simulink model "eVTOL_PX4_2023b"  (R2024b)
settings: Solver=ode4  StartTime=0  StopTime=inf  FixedStep=0.01  RelTol=1e-3
values from neighbouring files (symbols this model uses):
  aDl =     [initdata.mat]
  aDr =     [initdata.mat]
  aDyn =     [initdata.mat]
  Airport = init_airport('PHNL')    [initdata_HIL_eVTOL.m]
  aLat =     [initdata.mat]
  aLon =     [initdata.mat]
  D = Prop.D    [EOM_dt_MC.m]    (also in EOM_get_alf_dt_de_prop_evtol.m = CD * QS)
  dt0 = X(2)    [EOM_get_alf_dt_de_prop_evtol.m]    (also in initdata.mat = 0.258252593971; initdata_HIL_eVTOL.m = EOM_dt_MC)
  EAS0 = TAS0 / EAS2TAS    [initdata_HIL_eVTOL.m]
  FCS = init_FCS    [initdata_HIL_eVTOL.m]
  General = init_layoutdata    [EOM_dt_MC.m]    (also in build_optimized_CA.m; initdata.mat = ; initdata_HIL_eVTOL.m)
  h0 = Con(1)    [EOM_get_alf_dt_de_prop_evtol.m]    (also in initdata.mat = 450; initdata_HIL_eVTOL.m = 50)
  mass = Con(3)    [EOM_get_alf_dt_de_prop_evtol.m]    (also in initdata.mat = 2255.54; initdata_HIL_eVTOL.m = 7)
  Motor = init_motor_evtol    [EOM_dt_MC.m]    (also in initdata.mat = []; initdata_HIL_eVTOL.m)
  Prop = init_propeller_evtol_new    [EOM_dt_MC.m]    (also in initdata_HIL_eVTOL.m)
  R2D = 180/pi    (= 57.2957795131)    [EOM_get_alf_dt_de_prop_evtol.m]    (also in init_FCS.m; init_aerodata_evtol.m; init_airport.m; initdata.mat)
  SAMPLE_TIME = 0.01    [initdata_HIL_eVTOL.m]
  theta0 = -0.0510981441662    [initdata.mat]
undefined symbols (not defined in the file or in its folder): A1, aDa, aDe, aero, asbhl20env, B1, C1, de0, Earth, Environment, INIT_Data, InitData, Kd, Kp, magnitude, Newton, pProp, Raphson, Tc, WGS84
libraries: simulink_extras x63, vrlib x48, sharedtransform x28, simulink x22, slpidlib x20, sharedutil x20, matrix_library x18, aerolibwindfilters x12, aerolibobsolete x8, aerolibasang x8, aerolibatmos2 x6, aerolibfltsims x6
(part 3 of 17)

== system eVTOL_PX4_2023b/Subsystem2/airframe ==
  EnvmData : Inport
  prop : Inport  Port=2
  Act_surface : Inport  Port=3
  SW : Inport  Port=4
  6DoF (Euler Angles)1 : aerolibobsolete/6DoF (Euler Angles)  units=Metric (MKS)  mtype=Fixed  rep=Euler Angles  xme_0=InitData.Xe  Vm_0=InitData.Vb  eul_0=InitData.Euler+[0,0,0]/57.3  pm_0=InitData.pqr  mass_0=InitData.mass0  mass_e=0.5  mass_f=2.0  inertia=Mass.Inertial  inertia_e=eye(3)  inertia_f=2*eye(3)  k_quat=1.0
  Bus Creator : BusCreator  Inputs=25
  Constant3 : Constant  Value=mass
  Flight Conditions : Subsystem  AncestorBlock=asbhl20vehicle/Vehicle/Aerodynamic/DerivedConditions
      settings: LibrarySourceBlock=asbhl20vehicle/Vehicle/Aerodynamic/DerivedConditions
  Fly : Constant
  Gain : Gain  Gain=[1,1,1]
  Gain1 : Gain  Gain=[1,1,1]
  Product : Product
  Product1 : Product
  Switch2 : Switch  Criteria=u2 > Threshold  SaturateOnIntegerOverflow=off  InputSameDT=off
  force moment : Subsystem
  init : Constant  Value=0
  UAVData : Outport  VectorParamsAs1DForOutWhenUnconnected=off
  wires:
  prop/1 -> force moment/3(prop)
  6DoF (Euler Angles)1/1 -> Bus Creator/1  "Ve"
  6DoF (Euler Angles)1/2 -> Bus Creator/2  "Xe"
  6DoF (Euler Angles)1/8 -> Bus Creator/8  "Ab"
  6DoF (Euler Angles)1/7 -> Bus Creator/7  "pqr_dot"
  6DoF (Euler Angles)1/6 -> Bus Creator/6  "pqr"
  6DoF (Euler Angles)1/5 -> Bus Creator/5  "Vb"
  Act_surface/1 -> force moment/2(Act_surface)
  Bus Creator/1 -> UAVData/1, force moment/1(PlantData), Flight Conditions/2(PlantData)  "UAVData"
  EnvmData/1 -> Flight Conditions/1(EnvmData), force moment/4(EnvmData)
  Flight Conditions/6(Beta) -> Bus Creator/14  "beta"
  Flight Conditions/7(V) -> Bus Creator/15  "Va"
  Flight Conditions/9(pqrWind) -> Bus Creator/17  "pqrWind"
  Flight Conditions/10(Mach) -> Bus Creator/18  "mach"
  Flight Conditions/11(Qbar) -> Bus Creator/19  "Q"
  Flight Conditions/12(gamma) -> Bus Creator/20  "gamma"
  Flight Conditions/5(AlphaDot) -> Bus Creator/13  "alphaDot"
  6DoF (Euler Angles)1/4 -> Bus Creator/4  "DCM_be"
  Constant3/1 -> Bus Creator/25  "mass"
  Flight Conditions/13(chi) -> Bus Creator/21  "chi"
  Flight Conditions/14(Po) -> Bus Creator/22  "Po"
  Flight Conditions/15(To) -> Bus Creator/23  "To"
  Flight Conditions/16(g) -> Bus Creator/24  "g"
  force moment/1(Fb (X Y Z)) -> Gain/1
  force moment/2(M (L M N)) -> Gain1/1
  6DoF (Euler Angles)1/3 -> Bus Creator/3  "Euler"
  Product/1 -> 6DoF (Euler Angles)1/1
  Gain1/1 -> Product1/2
  Product1/1 -> 6DoF (Euler Angles)1/2
  Gain/1 -> Product/2
  Switch2/1 -> Product1/1, Product/1  "是否关闭力输出"
  Fly/1 -> Switch2/1
  SW/1 -> Switch2/2
  init/1 -> Switch2/3
  Flight Conditions/3(amsl) -> Bus Creator/11  "AMSL"
  Flight Conditions/2(lon_deg) -> Bus Creator/10  "lon_deg"
  Flight Conditions/1(lat_deg) -> Bus Creator/9  "lat_deg"
  Flight Conditions/4(Alpha) -> Bus Creator/12  "alpha"
  Flight Conditions/8(EAS) -> Bus Creator/16  "EAS"

== system eVTOL_PX4_2023b/UAV/Energy & Power ==
  UAVData : Inport
  ActData : Inport  Port=2
  Bus Creator : BusCreator  Inputs=8
  Bus Selector1 : BusSelector  OutputSignals=dt
  Bus Selector2 : BusSelector  OutputSignals=Va
  Constant : Constant
  Constant1 : Constant
  Constant2 : Constant  Value=8000
  Constant3 : Constant  Value=8000
  Constant4 : Constant  Value=500
  Constant5 : Constant  Value=500
  Gain : Gain  Gain=pProp.TDt
  Gain1 : Gain  Gain=pProp.TV
  Gain2 : Gain
  Gain3 : Gain
  Sum : Sum  Inputs=|++
  PropData : Outport  VectorParamsAs1DForOutWhenUnconnected=off
  wires:
  Constant2/1 -> Bus Creator/8  "rpm_r"
  Constant3/1 -> Bus Creator/5  "rpm_l"
  Gain3/1 -> Bus Creator/7  "T_r"
  Constant1/1 -> Bus Creator/6  "eta_prop_r"
  Bus Creator/1 -> PropData/1
  ActData/1 -> Bus Selector1/1
  Constant/1 -> Bus Creator/3  "eta_prop_l"
  Gain2/1 -> Bus Creator/4  "T_l"
  Bus Selector1/1 -> Gain/1  "<dt>"
  UAVData/1 -> Bus Selector2/1
  Bus Selector2/1 -> Gain1/1  "<Va>"
  Gain/1 -> Sum/1
  Gain1/1 -> Sum/2
  Sum/1 -> Gain3/1, Gain2/1  "T"
  Constant4/1 -> Bus Creator/1  "P_tot"
  Constant5/1 -> Bus Creator/2  "wh_remain"

== system eVTOL_PX4_2023b/UAV/Environment ==
  plane : Inport
  WindSpeed : Inport  Port=2
  Bus Creator : BusCreator  Inputs=8
  Bus Selector : BusSelector  OutputSignals=Xe,Ve,DCM_be
  COESA Atmosphere Model : aerolibatmos2/COESA Atmosphere Model  units=Metric (MKS)  spec=1976 COESA-extended U.S. Standard Atmosphere  model=Profile  profile_var=High temperature  profile_percent=1%  profile_alt=5 km (16404 ft)  envelope_var=High temperature  envelope_percent=1%  action=Warning
  Height : Selector  InputPortWidth=3  IndexOptions=Index vector (dialog)  Indices=[3]  OutputSizes=1
  Latitude : Constant  Value=40
  Terrain : Subsystem
  WGS84 Gravity Model : aerolibobsolete/WGS84 Gravity Model  model=WGS84 Taylor Series  units=Metric (MKS)  no_atmos=on  precessing=on  month=February  day=1  year=2000  no_centrifugal=on  action=None
  Wind Models : Subsystem
  z-->h : Abs
  Envm : Outport  InitialOutput=0  VectorParamsAs1DForOutWhenUnconnected=off
  wires:
  COESA Atmosphere Model/4 -> Bus Creator/7  "AirDensity"
  COESA Atmosphere Model/2 -> Bus Creator/5  "a"
  COESA Atmosphere Model/3 -> Bus Creator/6  "Po"
  COESA Atmosphere Model/1 -> Bus Creator/4  "To"
  Height/1 -> z-->h/1
  Bus Creator/1 -> Envm/1  "EnvmData"
  plane/1 -> Bus Selector/1
  z-->h/1 -> COESA Atmosphere Model/1, WGS84 Gravity Model/1, Wind Models/3(Altitude)
  Bus Selector/1 -> Terrain/1(Xe), Height/1  "<Xe>"
  Bus Selector/2 -> Wind Models/2(Ve)  "<Ve>"
  Bus Selector/3 -> Wind Models/4(DCM)  "<DCM_be>"
  Latitude/1 -> WGS84 Gravity Model/2
  WGS84 Gravity Model/1 -> Bus Creator/8  "g"
  Terrain/1(hground) -> Bus Creator/1  "hground"
  Wind Models/1(ug,vg,wg) -> Bus Creator/2
  Wind Models/2(pg,qg,rg) -> Bus Creator/3
  WindSpeed/1 -> Wind Models/1(WindSpeed)

== system eVTOL_PX4_2023b/UAV/airframe ==
  EnvmData : Inport
  PropData : Inport  Port=2
  ActData : Inport  Port=3
  SW : Inport  Port=4
  6DoF (Quaternion) : aerolibobsolete/6DoF (Euler Angles)  units=Metric (MKS)  mtype=Fixed  rep=Quaternion  xme_0=InitData.Xe  Vm_0=InitData.Vb  eul_0=InitData.Euler+[0,0,0]/57.3  pm_0=InitData.pqr  mass_0=General.mass  mass_e=0.5  mass_f=2.0  inertia=General.Inertia  inertia_e=eye(3)  inertia_f=2*eye(3)  k_quat=1.0
  Bus Creator1 : BusCreator  Inputs=25
  Constant3 : Constant  Value=General.mass
  Flight Conditions : Subsystem  AncestorBlock=asbhl20vehicle/Vehicle/Aerodynamic/DerivedConditions
  Fly : Constant
  Gain : Gain  Gain=[1,1,1]
  Gain1 : Gain  Gain=[1,1,1]
  Product : Product
  Product1 : Product
  Scope6 : Scope
  Switch2 : Switch  Criteria=u2 > Threshold  SaturateOnIntegerOverflow=off  InputSameDT=off
  force moment : Subsystem
  init : Constant  Value=0
  UAVData : Outport  VectorParamsAs1DForOutWhenUnconnected=off
  wires:
  PropData/1 -> force moment/3(EngineData_lo)
  6DoF (Quaternion)/1 -> Scope6/1, Bus Creator1/1  "Ve"
  6DoF (Quaternion)/2 -> Bus Creator1/2  "Xe"
  6DoF (Quaternion)/8 -> Bus Creator1/8  "Ab"
  6DoF (Quaternion)/7 -> Bus Creator1/7  "pqr_dot"
  6DoF (Quaternion)/6 -> Bus Creator1/6  "pqr"
  6DoF (Quaternion)/5 -> Bus Creator1/5  "Vb"
  ActData/1 -> force moment/2(ActData)
  Bus Creator1/1 -> UAVData/1, force moment/1(PlantData), Flight Conditions/2(PlantData)  "UAVData"
  EnvmData/1 -> force moment/4(EnvmData), Flight Conditions/1(EnvmData)
  Flight Conditions/4(Alpha) -> Bus Creator1/12  "alpha"
  Flight Conditions/6(Beta) -> Bus Creator1/14  "beta"
  Flight Conditions/7(V) -> Bus Creator1/15  "Va"
  Flight Conditions/9(pqrWind) -> Bus Creator1/17  "pqrWind"
  Flight Conditions/10(Mach) -> Bus Creator1/18  "mach"
  Flight Conditions/11(Qbar) -> Bus Creator1/19  "Q"
  Flight Conditions/12(gamma) -> Bus Creator1/20  "gamma"
  Flight Conditions/5(AlphaDot) -> Bus Creator1/13  "alphaDot"
  6DoF (Quaternion)/4 -> Bus Creator1/4  "DCM_be"
  Constant3/1 -> Bus Creator1/25  "mass"
  Flight Conditions/13(chi) -> Bus Creator1/21  "chi"
  Flight Conditions/14(Po) -> Bus Creator1/22  "Po"
  Flight Conditions/15(To) -> Bus Creator1/23  "To"
  Flight Conditions/16(g) -> Bus Creator1/24  "g"
  force moment/1(Fb (X Y Z)) -> Gain/1
  force moment/2(M (L M N)) -> Gain1/1
  6DoF (Quaternion)/3 -> Bus Creator1/3  "Euler"
  init/1 -> Switch2/3
  Product/1 -> 6DoF (Quaternion)/1
  Gain1/1 -> Product1/2
  Product1/1 -> 6DoF (Quaternion)/2
  Fly/1 -> Switch2/1
  Switch2/1 -> Product/1, Product1/1
  Gain/1 -> Product/2
  SW/1 -> Switch2/2
  Flight Conditions/1(lat_deg) -> Bus Creator1/9  "lat_deg"
  Flight Conditions/2(lon_deg) -> Bus Creator1/10  "lon_deg"
  Flight Conditions/3(amsl) -> Bus Creator1/11  "AMSL"
  Flight Conditions/8(EAS) -> Bus Creator1/16  "EAS"

== system eVTOL_PX4_2023b/hil_state_quaternion_pack1/payload_hil_state_quaternion ==
  time_s : Inport
  DCM_be : Inport  Port=2
  body_rate : Inport  Port=3
  latlon_deg : Inport  Port=4
  amsl : Inport  Port=5
  Ve : Inport  Port=6
  ab : Inport  Port=7
  EAS : Inport  Port=8
  TAS : Inport  Port=9
  1g : Constant  Value=[0,0,9.8]
  Bus Creator1 : BusCreator  Inputs=16
  Data Type Conversion10 : DataTypeConversion  OutDataTypeStr=int32  SaturateOnIntegerOverflow=off  RndMeth=Floor
  Data Type Conversion11 : DataTypeConversion  OutDataTypeStr=int32  SaturateOnIntegerOverflow=off  RndMeth=Floor
  Data Type Conversion{12..17} (6 alike) : DataTypeConversion  OutDataTypeStr=int16  SaturateOnIntegerOverflow=off  RndMeth=Floor
  Data Type Conversion18 : DataTypeConversion  OutDataTypeStr=uint64  SaturateOnIntegerOverflow=off  RndMeth=Floor
  Data Type Conversion2 : DataTypeConversion  OutDataTypeStr=uint16  SaturateOnIntegerOverflow=off  RndMeth=Floor
  Data Type Conversion{6..8,20} (4 alike) : DataTypeConversion  OutDataTypeStr=single  SaturateOnIntegerOverflow=off  RndMeth=Floor
  Data Type Conversion3 : DataTypeConversion  OutDataTypeStr=uint16  SaturateOnIntegerOverflow=off  RndMeth=Floor
  Data Type Conversion9 : DataTypeConversion  OutDataTypeStr=int32  SaturateOnIntegerOverflow=off  RndMeth=Floor
  Demux : Demux  Outputs=3
  Demux2 : Demux  Outputs=3
  Demux4 : Demux  Outputs=2
  Demux5 : Demux  Outputs=3
  Direction Cosine Matrix to Quaternions : sharedtransform/Direction Cosine Matrix  to Quaternions  aMode=0  action=None  tolerance=eps(2)
  Gain : Gain  Gain=100
  Gain1 : Gain  Gain=1e2
  Gain2 : Gain  Gain=1e7
  Gain3 : Gain  Gain=1e6
  Gain4 : Gain  Gain=1e3
  Gain5 : Gain  Gain=1e2
  Gain6 : Gain  Gain=1e2
  Gain7 : Gain  Gain=100
  Gain8 : Gain  Gain=100
  Manual Switch : ManualSwitch
  Product : Product  Multiplication=Matrix(*)
  Sum : Sum  Inputs=+-|
  Payload : Outport
  wires:
  Data Type Conversion11/1 -> Bus Creator1/8  "alt"
  Data Type Conversion14/1 -> Bus Creator1/11  "vz"
  Demux2/2 -> Data Type Conversion7/1  "pitchspeed"
  Data Type Conversion7/1 -> Bus Creator1/4  "pitchspeed"
  Data Type Conversion16/1 -> Bus Creator1/15  "yacc"
  Demux4/2 -> Data Type Conversion10/1  "lon"
  Gain5/1 -> Demux/1
  Demux/2 -> Data Type Conversion13/1  "vy"
  Demux/3 -> Data Type Conversion14/1  "vz"
  Demux2/3 -> Data Type Conversion8/1  "yawspeed"
  Data Type Conversion10/1 -> Bus Creator1/7  "lon"
  Gain2/1 -> Demux4/1  "lon"
  Data Type Conversion13/1 -> Bus Creator1/10  "vy"
  amsl/1 -> Gain4/1
  Data Type Conversion9/1 -> Bus Creator1/6  "lat"
  Data Type Conversion17/1 -> Bus Creator1/16  "zacc"
  Data Type Conversion12/1 -> Bus Creator1/9  "vx"
  time_s/1 -> Gain3/1
  Demux2/1 -> Data Type Conversion6/1  "rollspeed"
  Demux4/1 -> Data Type Conversion9/1  "lat"
  Gain3/1 -> Data Type Conversion18/1
  Data Type Conversion18/1 -> Bus Creator1/1  "time_usec"
  body_rate/1 -> Demux2/1
  Gain4/1 -> Data Type Conversion11/1
  Data Type Conversion15/1 -> Bus Creator1/14  "xacc"
  [accel_meas] -> Demux5/1
  Data Type Conversion6/1 -> Bus Creator1/3  "rollspeed"
  Demux/1 -> Data Type Conversion12/1  "vx"
  latlon_deg/1 -> Gain2/1
  DCM_be/1 -> Product/1, Direction Cosine Matrix to Quaternions/1
  Data Type Conversion8/1 -> Bus Creator1/5  "yawspeed"
  Bus Creator1/1 -> Payload/1  "Payload"
  Ve/1 -> Gain5/1
  Direction Cosine Matrix to Quaternions/1 -> Data Type Conversion20/1
  TAS/1 -> Gain1/1
  Gain1/1 -> Data Type Conversion3/1
  Data Type Conversion20/1 -> Bus Creator1/2  "attitude_quaternion"
  Data Type Conversion2/1 -> Bus Creator1/12  "ind_airspeed"
  Data Type Conversion3/1 -> Bus Creator1/13  "true_airspeed"
  Demux5/3 -> Gain/1  "zacc"
  Gain/1 -> Data Type Conversion17/1  "zacc(mG)"
  Demux5/1 -> Gain8/1  "xacc"
  Demux5/2 -> Gain7/1  "yacc"
  Gain8/1 -> Data Type Conversion15/1  "xacc(mG)"
  Gain7/1 -> Data Type Conversion16/1  "yacc(mG)"
  EAS/1 -> Gain6/1
  Gain6/1 -> Data Type Conversion2/1
  Product/1 -> Sum/2
  1g/1 -> Product/2
  ab/1 -> Manual Switch/1, Sum/1  "acceleration"
  Sum/1 -> Manual Switch/2  "specific force"
  Manual Switch/1 -> [accel_meas]

== system eVTOL_PX4_2023b/FCS/FW/Flare ==
  note: In my paper:
      | KHDot_Flare=0.024
      | KH_Flare=0.037
  H : Inport
  HDot : Inport  Port=2
  Enable : EnablePort
  Divide : Product  Inputs=*/
  Divide1 : Product  Inputs=**
  Gain : Gain
  HDot_Flare V=11 : Constant  Value=-0.57
  HDot_Flare V=12 : Constant  Value=-0.62
  HDot_TD : Constant  Value=-0.2
  H_Flare : Constant  Value=501.4
  H_TD : Constant  Value=500.4
  Integrator : Integrator
  KHDot_flare : Gain  Gain=0.6
  KH_flare : Gain  Gain=1.2
  Sum : Sum  Inputs=|++
  Sum1 : Sum  Inputs=|++
  Sum2 : Sum  Inputs=|+-
  Sum3 : Sum  Inputs=-+|
  Sum4 : Sum  Inputs=|+-
  Sum5 : Sum  Inputs=|+-
  Sum6 : Sum  Inputs=|++
  Transfer Fcn : TransferFcn  Numerator=[10 3]  Denominator=[1 3]
  dHdot Scope : Scope  NumInputPorts=2
  glide angle : Constant  Value=-3/57.3
  thetac : Outport  VectorParamsAs1DForOutWhenUnconnected=off
  wires:
  HDot/1 -> dHdot Scope/2, Sum3/1
  Sum3/1 -> KH_flare/1, KHDot_flare/1  "dHDot"
  Divide/1 -> Gain/1
  KH_flare/1 -> Integrator/1
  Sum/1 -> Sum6/1, Transfer Fcn/1
  Sum1/1 -> dHdot Scope/1, Sum3/2  "HDot_c"
  KHDot_flare/1 -> Sum/1
  Integrator/1 -> Sum/2
  Transfer Fcn/1 -> ?  "thetac"
  H_TD/1 -> Sum5/2, Sum4/2
  HDot_Flare V=11/1 -> Sum2/1
  H/1 -> Sum5/1
  Sum2/1 -> Divide/1
  HDot_TD/1 -> Sum2/2, Sum1/2
  Sum4/1 -> Divide/2
  H_Flare/1 -> Sum4/1
  Gain/1 -> Divide1/1
  Divide1/1 -> Sum1/1
  Sum5/1 -> Divide1/2
  Sum6/1 -> thetac/1
  glide angle/1 -> Sum6/2

== system eVTOL_PX4_2023b/FCS/FW/L1 guidance ==
  L1Mod : Inport
  L1 : Inport  Port=2
  R_circle : Inport  Port=3
  SensorData : Inport  Port=4
  NAVData : Inport  Port=5
  Bus Selector1 : BusSelector  OutputSignals=d,chi_WP
  Bus Selector3 : BusSelector  OutputSignals=Ve,chi
  Divide : Product  Inputs=*/
  Divide1 : Product  Inputs=*/
  Divide2 : Product  Inputs=***
  Divide3 : Product  Inputs=/*
  Divide4 : Product  Inputs=*/
  Dot Product : DotProduct  OutDataTypeStr=Inherit: Inherit via internal rule
  Gain : Gain  Gain=2
  Gain1 : Gain
  Gain2 : Gain  Gain=1/2
  Gain3 : Gain
  Multiport Switch : MultiPortSwitch  Inputs=2  SaturateOnIntegerOverflow=off  InputSameDT=off
  Radians to Degrees1 : simulink_extras/Transformations/Radians to Degrees
  Radians to Degrees2 : simulink_extras/Transformations/Radians to Degrees
  Radians to Degrees6 : simulink_extras/Transformations/Radians to Degrees
  Sqrt : Sqrt
  Sum : Sum  Inputs=|-+
  Sum1 : Sum  Inputs=|-+
  Sum2 : Sum  Inputs=|++
  Trigonometric Function : Trigonometry  Operator=asin
  Trigonometric Function1 : Trigonometry
  Trigonometric Function2 : Trigonometry  Operator=atan
  V : Scope
  "[+-0.7072]" : Saturate  UpperLimit=0.7072  LowerLimit=-0.7072
  ay : Scope
  chi_tr scp : Scope
  d scp : Scope
  eta1 scp : Scope
  eta{2..8} (7 alike) : Scope
  g : Constant  Value=9.8
  phic scp : Scope
  yc : Constant  Value=0
  phi_c : Outport  VectorParamsAs1DForOutWhenUnconnected=off
  eta1 : Outport  Port=2  VectorParamsAs1DForOutWhenUnconnected=off
  wires:
  [d] -> Sum/1
  Sum/1 -> d scp/1, Gain1/1  "d"
  L1/1 -> Gain2/1, eta5/1, Divide1/2, Divide/2
  Divide/1 -> "[+-0.7072]"/1
  Trigonometric Function/1 -> Sum2/1, Radians to Degrees2/1, eta1/1  "eta1"
  Trigonometric Function1/1 -> eta3/1, Multiport Switch/3  "sin(eta)_line"
  Divide1/1 -> eta4/1, Gain/1
  Gain/1 -> Divide2/3
  [V] -> Divide2/2, Divide2/1
  Divide2/1 -> Divide3/2, ay/1  "ay"
  g/1 -> Divide3/1
  Divide3/1 -> Trigonometric Function2/1
  Trigonometric Function2/1 -> phi_c/1, Radians to Degrees6/1
  Gain1/1 -> Divide/1
  Sum1/1 -> Gain3/1  "eta2"
  Sum2/1 -> Trigonometric Function1/1
  Multiport Switch/1 -> eta6/1, Divide1/1
  Gain2/1 -> Divide4/1
  Divide4/1 -> eta8/1, Multiport Switch/2  "sin(eta)_circle"
  R_circle/1 -> Divide4/2
  [chi] -> Sum1/1  "eta2"
  [chi_WP] -> Radians to Degrees1/1, Sum1/2
  L1Mod/1 -> Multiport Switch/1, eta7/1
  Radians to Degrees6/1 -> phic scp/1
  Radians to Degrees1/1 -> chi_tr scp/1
  Bus Selector1/1 -> [d]  "<d>"
  Bus Selector3/1 -> Dot Product/1, Dot Product/2  "<Ve>"
  NAVData/1 -> Bus Selector1/1
  Bus Selector3/2 -> [chi]  "<chi>"
  Bus Selector1/2 -> [chi_WP]  "<chi_WP>"
  SensorData/1 -> Bus Selector3/1
  yc/1 -> Sum/2
  Dot Product/1 -> Sqrt/1
  Sqrt/1 -> V/1, [V]
  Gain3/1 -> Sum2/2, eta2/1  "eta2"
  "[+-0.7072]"/1 -> Trigonometric Function/1
  Radians to Degrees2/1 -> eta1 scp/1

== system eVTOL_PX4_2023b/FCS/FW/TECS ==
  FCSCMD : Inport
  SensorData : Inport  Port=2
  NAVCMD : Inport  Port=3
  Bus Selector1 : BusSelector  OutputSignals=Hc,TASc
  Bus Selector6 : BusSelector  OutputSignals=LonMod,Hc,Vc_TAS
  Bus Selector7 : BusSelector  OutputSignals=LLA_deg,Va
  Gain1 : Gain  Commented=on  Gain=-1
  Hc : Step  Commented=on  Time=20  Before=h0  After=h0+10  SampleTime=0
  Hc WP : Scope
  Manual Switch : ManualSwitch
  Manual Switch1 : ManualSwitch
  Selector3 : Selector  InputPortWidth=3  IndexOptions=Index vector (dialog)  Indices=3  OutputSizes=1
  Selector4 : Selector  Commented=on  InputPortWidth=3  IndexOptions=Index vector (dialog)  Indices=2  OutputSizes=1
  TECS PX4 & AP201 : Subsystem
  VC : Step  Commented=on  Time=0  Before=EAS0  After=EAS0  SampleTime=0
  Vc WP : Scope
  Vc_TAS scp : Scope
  thetac : Outport  VectorParamsAs1DForOutWhenUnconnected=off
  dt : Outport  Port=2  VectorParamsAs1DForOutWhenUnconnected=off
  wires:
  Selector3/1 -> TECS PX4 & AP201/2(h)
  Bus Selector6/1 -> TECS PX4 & AP201/1(LonMod)  "<LonMod>"
  SensorData/1 -> Bus Selector7/1
  Bus Selector7/2 -> TECS PX4 & AP201/3(V)  "<Va>"
  Selector4/1 -> Gain1/1
  Bus Selector7/1 -> Selector3/1  "<LLA_deg>"
  FCSCMD/1 -> Bus Selector6/1
  NAVCMD/1 -> Bus Selector1/1
  Manual Switch1/1 -> TECS PX4 & AP201/4(hc)
  Bus Selector6/3 -> Manual Switch/1  "<Vc_TAS>"
  Bus Selector1/2 -> Manual Switch/2, Vc WP/1  "<TASc>"
  Bus Selector1/1 -> Manual Switch1/2, Hc WP/1  "<Hc>"
  Bus Selector6/2 -> Manual Switch1/1  "<Hc>"
  TECS PX4 & AP201/2(thetac) -> thetac/1
  TECS PX4 & AP201/1(dt) -> dt/1
  Manual Switch/1 -> Vc_TAS scp/1, TECS PX4 & AP201/5(Vc)

== system eVTOL_PX4_2023b/FCS/FW/V hold//control ==
  note: VMod:
      | 1-cruise throt
      | 2-max throt
      | 3-min throt
      | 4-TECS
      | 5-Flare dt Fade
  CMDData : Inport
  SensorData : Inport  Port=2
  dt : Inport  Port=3
  Add : Sum
  Bus Selector1 : BusSelector  OutputSignals=Va
  Bus Selector4 : BusSelector  OutputSignals=VMod,Vc_TAS
  Compare To Constant : simulink/Logic and Bit Operations/Compare To Constant  relop===  const=1  OutDataTypeStr=uint8  ZeroCross=off
  Compare To Constant1 : simulink/Logic and Bit Operations/Compare To Constant  relop===  const=5  OutDataTypeStr=uint8  ZeroCross=off
  From1 : From  Commented=on  GotoTag=dtTrim  TagVisibility=scoped
      settings: CloseFcn=tagdialog Close
  From8 : From  Commented=on  GotoTag=dtTrim  TagVisibility=scoped
      settings: CloseFcn=tagdialog Close
  Multiport Switch : MultiPortSwitch  Inputs=5  SaturateOnIntegerOverflow=off  InputSameDT=off
  Saturation : Saturate  UpperLimit=FCS.dt_max  LowerLimit=FCS.dt_min
  Saturation Dynamic : simulink/Discontinuities/Saturation Dynamic  Commented=on  OutMin=[]  OutMax=[]  OutDataTypeStr=Inherit: Same as second input  OutDataType=fixdt(1, 16)  OutScaling=2^-10  DoSatur=off
  Saturation1 : Saturate  UpperLimit=1.4  LowerLimit=-1.4
  Subsystem3 : Subsystem
  dt Fade at 0.1 / sec : Subsystem  TreatAsAtomicUnit=on
  dt=0 : Constant  Value=0
  dt=1 : Constant
  dtTrim : Constant  Value=0
  dvbar scp : Scope
  dvbar scp1 : Scope
  getV_bar : Subsystem
  dt cmd : Outport  VectorParamsAs1DForOutWhenUnconnected=off
  wires:
  Saturation/1 -> dt cmd/1  "dt"
  Bus Selector4/1 -> Compare To Constant1/1, Compare To Constant/1, Multiport Switch/1  "<VMod>"
  Compare To Constant/1 -> Subsystem3/1(VMod)
  dt=1/1 -> Multiport Switch/3
  From8/1 -> ?
  Subsystem3/1(dt_cmd) -> Saturation1/1, dvbar scp1/1
  Saturation1/1 -> dvbar scp/1, Multiport Switch/2
  Bus Selector4/2 -> getV_bar/2(V_c)  "<Vc_TAS>"
  getV_bar/1(V_bar) -> Subsystem3/2(dvbar)
  dt=0/1 -> Multiport Switch/6, Multiport Switch/4
  Compare To Constant1/1 -> dt Fade at 0.1 / sec/Enable
  Multiport Switch/1 -> dt Fade at 0.1 / sec/1(dt_ini), Saturation/1
  CMDData/1 -> Bus Selector4/1
  SensorData/1 -> Bus Selector1/1
  Bus Selector1/1 -> getV_bar/1(V)  "<Va>"
  dtTrim/1 -> Add/2
  dt/1 -> Add/1
  Add/1 -> Multiport Switch/5

== system eVTOL_PX4_2023b/FCS/FW/WayPoint Nav CMD ==
  note: FlightMod
      | 1-Ready
      | 2-TakeOff
      | 3-PullUp
      | 4-Climb
      | 5-Cruise, 5.1-circle, 5.2-line
      | 6-Return
      | 7-Approach
      | 8-Flare
      | 9-TouchDown
      | 10-Taxi
      | 11-GoAround
      | 12-Parachute
  SensorData : Inport
  Enable : EnablePort
  Bus Creator2 : BusCreator  Inputs=10
  Bus Selector3 : BusSelector  Commented=on  OutputSignals=IMUData.GPS_ENU,BaroData.V,BaroData.Ha
  Constant : Constant  Value=450
  Constant1 : Constant  Value=EAS0
  Constant2 : Constant  Commented=on  Value=1000
  Constant3 : Constant  Value=0
  Constant4 : Constant  Commented=on  Value=1000
  Constant5 : Constant  Value=0
  Constant6 : Constant  Commented=on  Value=0
  Constant7 : Constant  Value=450
  From : From  Commented=on  GotoTag=DS
  From3 : From  Commented=on  GotoTag=d_rem
  Gain : Gain  Gain=1/1.225
  Goto : Goto  Commented=on  GotoTag=DS
  Goto3 : Goto  Commented=on  GotoTag=d_rem
  Goto7 : Goto  Commented=on  GotoTag=dh_2traj
  ISA Atmosphere Model : aerolibatmos2/ISA Atmosphere Model  useExtended=off  action=Warning  custom=off  viscosityOut=off  g=9.80665  gamma=1.4  R=287.0531  L=0.0065  h_trop=11000  h_strat=20000  rho0=1.225  P0=101325  T0=288.15  h0=0
  Mission_ID : Constant  Value=0
  Mux1 : Mux  Inputs=6
  Product : Product  Inputs=*/
  Selector1 : Selector  Commented=on  InputPortWidth=3  IndexOptions=Index vector (dialog)  Indices=2  OutputSizes=1
  Selector2 : Selector  Commented=on  InputPortWidth=3  IndexOptions=Index vector (dialog)  Indices=1  OutputSizes=1
  Selector3 : Selector  Commented=on  InputPortWidth=3  IndexOptions=Index vector (dialog)  Indices=3  OutputSizes=1
  Sqrt : Sqrt
  Terminator : Terminator
  Terminator1 : Terminator
  Terminator2 : Terminator
  WP# : Constant
  NAVCMD : Outport  VectorParamsAs1DForOutWhenUnconnected=off
  wires:
  WP#/1 -> Mux1/5
  From/1 -> Bus Creator2/6  "DS"
  [d] -> Bus Creator2/4  "d"
  From3/1 -> Bus Creator2/5  "d_rem"
  Selector2/1 -> Mux1/2  "lon"
  Selector1/1 -> Mux1/1  "lat"
  Mux1/1 -> Bus Creator2/1  "UAVPos"
  [chi_WP] -> Bus Creator2/7  "chi_WP"
  Bus Creator2/1 -> NAVCMD/1
  [Hc] -> Bus Creator2/8  "Hc"
  [EASc] -> Bus Creator2/9  "EASc"
  SensorData/1 -> Bus Selector3/1
  Bus Selector3/2 -> Mux1/4  "<V>"
  Bus Selector3/1 -> Selector2/1, Selector3/1, Selector1/1  "<GPS_ENU>"
  Selector3/1 -> Mux1/3  "h"
  Constant2/1 -> Goto/1
  Constant3/1 -> [chi_WP]
  Constant5/1 -> [d]
  Constant4/1 -> Goto3/1
  Constant7/1 -> [H_WPB]
  Constant1/1 -> [EASc]
  Constant6/1 -> Goto7/1
  Constant/1 -> [Hc]
  Mission_ID/1 -> Mux1/6
  Bus Selector3/3 -> ISA Atmosphere Model/1  "<Ha>"
  ISA Atmosphere Model/1 -> Terminator/1
  ISA Atmosphere Model/2 -> Terminator1/1
  ISA Atmosphere Model/3 -> Terminator2/1
  ISA Atmosphere Model/4 -> [rho]
  [rho] -> Gain/1
  Gain/1 -> Sqrt/1
  [EASc] -> Product/1  "TASc"
  Sqrt/1 -> Product/2
  Product/1 -> [TASc]
  [TASc] -> Bus Creator2/10  "TASc"

== system eVTOL_PX4_2023b/FCS/FW/alpha limit ==
  alpha : Inport
  Add2 : Sum  Inputs=-+
  Compare To Constant : simulink/Logic and Bit Operations/Compare To Constant  relop=>=  const=0  OutDataTypeStr=uint8  ZeroCross=off
  Lookup Table : Lookup  InputValues=[7, 7.5, 8.0] ./57.3  Table=[-50, -120,-250]  SaturateOnIntegerOverflow=off
  Product : Product  RndMeth=Zero
  Saturation1 : Saturate  UpperLimit=inf  LowerLimit=0
  Scope1 : Scope
  Scope2 : Scope
  Subsystem : Subsystem
  limit alpha : Constant  Value=7/57.3
  de : Outport  VectorParamsAs1DForOutWhenUnconnected=off
  wires:
  Subsystem/1(Out1) -> Scope1/1, de/1
  limit alpha/1 -> Add2/1
  alpha/1 -> Add2/2, Lookup Table/1
  Add2/1 -> Compare To Constant/1, Saturation1/1, Scope2/1
  Saturation1/1 -> Product/1
  Compare To Constant/1 -> Subsystem/Enable
  Product/1 -> Subsystem/1(In1)
  Lookup Table/1 -> Product/2

== system eVTOL_PX4_2023b/FCS/FW/phi hold&control ==
  phic : Inport
  SensorData : Inport  Port=2
  Bus Selector1 : BusSelector  OutputSignals=Euler,pqr,Ab,Va
  Divide : Product  Inputs=*/
  Gain : Gain
  Gain1 : Gain  Gain=-1
  Integrator : Integrator  Commented=on  LimitOutput=on  UpperSaturationLimit=0.2  LowerSaturationLimit=-0.2
  Kp_dd : Gain  Commented=on  Gain=0.05
  Kphi : Gain  Gain=0.25
  Kpi_dd : Gain  Commented=on  Gain=0.005
  Kr1 : Gain  Gain=9.8
  Kr2 : Gain  Gain=0.3
  PID Controller : slpidlib/PID Controller  Controller=PI  Form=Parallel  TimeDomain=Continuous-time  UseExternalTs=off  SampleTime=-1  IntegratorMethod=Forward Euler  FilterMethod=Forward Euler  ControllerParametersSource=internal  P=0.025  I=0005  UseKiTs=off  D=0  N=100  UseFilter=on  TunerSelectOption=Transfer Function Based (PID Tuner App)  InitialConditionSource=internal  InitialConditionForIntegrator=0  InitialConditionForFilter=0  DifferentiatorICPrevScaledInput=0  ExternalReset=none  TrackingMode=off  Kt=1  LimitOutput=on  SatLimitsSource=internal  UpperSaturationLimit=25/57.3  LowerSaturationLimit=-25/57.3  LinearizeAsGain=on  AntiWindupMode=none  Kb=1  LimitIntegrator=off  UpperIntegratorSaturationLimit=inf  LowerIntegratorSaturationLimit=-inf  POutMin=[]  POutMax=[]  IOutMin=[]  IOutMax=[]  DOutMin=[]  DOutMax=[]  NOutMin=[]  NOutMax=[]  SumOutMin=[]  SumOutMax=[]  SaturationOutMin=[]  SaturationOutMax=[]  PParamMin=[]  PParamMax=[]  IParamMin=[]  IParamMax=[]  DParamMin=[]  DParamMax=[]  NParamMin=[]  NParamMax=[]  KbParamMin=[]  KbParamMax=[]  KtParamMin=[]  KtParamMax=[]  KbOutMin=[]  KbOutMax=[]  KtOutMin=[]  KtOutMax=[]  IntegratorOutMin=[]  IntegratorOutMax=[]  FilterOutMin=[]  FilterOutMax=[]  SumI1OutMin=[]  SumI1OutMax=[]  SumI2OutMin=[]  SumI2OutMax=[]  SumI3OutMin=[]  SumI3OutMax=[]  SumI4OutMin=[]  SumI4OutMax=[]  SumDOutMin=[]  SumDOutMax=[]  DifferentiatorOutMin=[]  DifferentiatorOutMax=[]  FilterDiffOutCoefMin=[]  FilterDiffOutCoefMax=[]  ReciprocalOutMin=[]  ReciprocalOutMax=[]  SumDenOutMin=[]  SumDenOutMax=[]  SumNumOutMin=[]  SumNumOutMax=[]  DivideOutMin=[]  DivideOutMax=[]  UdiffTsProdOutMin=[]  UdiffTsProdOutMax=[]  NTsProdOutMin=[]  NTsProdOutMax=[]  UintegralTsProdOutMin=[]  UintegralTsProdOutMax=[]  UngainTsProdOutMin=[]  UngainTsProdOutMax=[]  ClampingZeroOutDataTypeStr=Inherit: Inherit via back propagation  ClampingZeroOutMin=[]  ClampingZeroOutMax=[]  FilterDenConstantOutDataTypeStr=Inherit: Inherit via back propagation  FilterDenConstantOutMin=[]  FilterDenConstantOutMax=[]  PCopyOutDataTypeStr=Inherit: Inherit via back propagation  PCopyOutMin=[]  PCopyOutMax=[]  NCopyOutDataTypeStr=Inherit: Inherit via back propagation  NCopyOutMin=[]  NCopyOutMax=[]  IntegratorContinuousStateAttributes=''  IntegratorStateMustResolveToSignalObject=off  IntegratorRTWStateStorageClass=Auto  FilterContinuousStateAttributes=''  FilterStateMustResolveToSignalObject=off  FilterRTWStateStorageClass=Auto  ParallelPVariant=InternalParameters  IdealPVariant=Disabled  IVariant=InternalParameters  DVariant=Disabled  IntegratorVariant=Continuous  SatVariant=Enabled  AWVariant=Passthrough  PCopyVariant=Disabled  TRVariant=Disabled  FdbkBlocksVariant=Forward  IdealPFdbkVariant=Disabled  SatFdbkVariant=Disabled  DerivativeFilterVariant=Disabled  NVariant=Disabled  NCopyVariant=Disabled_SignalSpec  FilterICVariant=Disabled  IntegratorICVariant=InternalICs  ExternalResetVariant=Disabled  TRSumVariant=Passthrough  SumFdbkVariant=Disabled  SumVariant=Sum_PI  TsampFilterVariant=InternalTs  TsampNgainVariant=Passthrough  TsampIntegralVariant=Disabled_SignalSpec  ExternalSaturationOutDataTypeStr=Inherit: Same as second input
  Radians to Degrees1 : simulink_extras/Transformations/Radians to Degrees
  Saturation : Saturate  UpperLimit=inf  LowerLimit=1
  Scope : Scope
  Scope1 : Scope
  Selector1 : Selector  InputPortWidth=3  IndexOptions=Index vector (dialog)  Indices=1  OutputSizes=1
  Selector2 : Selector  InputPortWidth=3  IndexOptions=Index vector (dialog)  Indices=1  OutputSizes=1
  Selector3 : Selector  InputPortWidth=3  IndexOptions=Index vector (dialog)  Indices=3  OutputSizes=1
  Selector4 : Selector  InputPortWidth=3  IndexOptions=Index vector (dialog)  Indices=2  OutputSizes=1
  Sum1 : Sum  Inputs=|+-
  Sum2 : Sum  Commented=on  Inputs=|++
  Sum4 : Sum  Inputs=|+-
  Sum5 : Sum  Inputs=|+-
  Tan : Trigonometry  Operator=tan
  da scp : Scope
  da : Outport  VectorParamsAs1DForOutWhenUnconnected=off
  dr : Outport  Port=2  VectorParamsAs1DForOutWhenUnconnected=off
  wires:
  phic/1 -> [phic]
  SensorData/1 -> Bus Selector1/1
  Bus Selector1/1 -> Selector1/1  "<Euler>"
  Selector1/1 -> [phi]
  Bus Selector1/2 -> Selector3/1, Selector2/1  "<pqr>"
  Selector2/1 -> [p]
  Selector3/1 -> [r]
  Bus Selector1/3 -> Selector4/1  "<Ab>"
  Selector4/1 -> [ay]
  [phic] -> Sum5/1
  [r] -> Kr2/1
  [p] -> Sum4/1
  Kr2/1 -> Sum1/1
  Integrator/1 -> Sum2/2
  Radians to Degrees1/1 -> da scp/1
  Kphi/1 -> Sum4/2  "pc"
  [phi] -> Sum5/2
  Kpi_dd/1 -> Integrator/1
  Sum4/1 -> Scope/1, PID Controller/1
  Sum5/1 -> Scope1/1, Kphi/1
  Kp_dd/1 -> Sum2/1
  [phi] -> Tan/1
  Tan/1 -> Kr1/1
  Bus Selector1/4 -> [Va]  "<Va>"
  Kr1/1 -> Divide/1
  Saturation/1 -> Divide/2
  [Va] -> Saturation/1
  Divide/1 -> Sum1/2
  Gain/1 -> Radians to Degrees1/1, da/1
  Sum1/1 -> Gain1/1
  Gain1/1 -> dr/1
  PID Controller/1 -> Gain/1

== system eVTOL_PX4_2023b/FCS/FW/theta hold&control ==
  note: LonMod:
      | 1-theta hold
      | 2-height hold
      | 3-gamma control
      | 4-landing flare control
      | 5-TakeOff
  CMDData : Inport
  SensorData : Inport  Port=2
  thetac : Inport  Port=3
  Add1 : Sum  Inputs=|-+
  Add2 : Sum  Inputs=|+-
  Add4 : Sum  Commented=on
  Bus Selector1 : BusSelector  OutputSignals=LonMod
  Bus Selector2 : BusSelector  OutputSignals=Euler,pqr
  Constant : Constant  Value=0
  Data Type Conversion : DataTypeConversion  OutDataTypeStr=boolean  SaturateOnIntegerOverflow=off  RndMeth=Floor
  Integrator : Integrator  Commented=on  ExternalReset=either  LimitOutput=on  UpperSaturationLimit=5  LowerSaturationLimit=-5
  Memory : Memory
  OMEGA : Gain  Gain=2
  PID Controller : slpidlib/PID Controller  Controller=PI  Form=Parallel  TimeDomain=Continuous-time  UseExternalTs=off  SampleTime=-1  IntegratorMethod=Forward Euler  FilterMethod=Forward Euler  ControllerParametersSource=internal  P=0.5  I=0.02  UseKiTs=off  D=0  N=100  UseFilter=on  TunerSelectOption=Transfer Function Based (PID Tuner App)  InitialConditionSource=internal  InitialConditionForIntegrator=0  InitialConditionForFilter=0  DifferentiatorICPrevScaledInput=0  ExternalReset=either  TrackingMode=off  Kt=1  LimitOutput=on  SatLimitsSource=internal  UpperSaturationLimit=25/57.3  LowerSaturationLimit=-25/57.3  LinearizeAsGain=on  AntiWindupMode=clamping  Kb=1  LimitIntegrator=off  UpperIntegratorSaturationLimit=inf  LowerIntegratorSaturationLimit=-inf  POutMin=[]  POutMax=[]  IOutMin=[]  IOutMax=[]  DOutMin=[]  DOutMax=[]  NOutMin=[]  NOutMax=[]  SumOutMin=[]  SumOutMax=[]  SaturationOutMin=[]  SaturationOutMax=[]  PParamMin=[]  PParamMax=[]  IParamMin=[]  IParamMax=[]  DParamMin=[]  DParamMax=[]  NParamMin=[]  NParamMax=[]  KbParamMin=[]  KbParamMax=[]  KtParamMin=[]  KtParamMax=[]  KbOutMin=[]  KbOutMax=[]  KtOutMin=[]  KtOutMax=[]  IntegratorOutMin=[]  IntegratorOutMax=[]  FilterOutMin=[]  FilterOutMax=[]  SumI1OutMin=[]  SumI1OutMax=[]  SumI2OutMin=[]  SumI2OutMax=[]  SumI3OutMin=[]  SumI3OutMax=[]  SumI4OutMin=[]  SumI4OutMax=[]  SumDOutMin=[]  SumDOutMax=[]  DifferentiatorOutMin=[]  DifferentiatorOutMax=[]  FilterDiffOutCoefMin=[]  FilterDiffOutCoefMax=[]  ReciprocalOutMin=[]  ReciprocalOutMax=[]  SumDenOutMin=[]  SumDenOutMax=[]  SumNumOutMin=[]  SumNumOutMax=[]  DivideOutMin=[]  DivideOutMax=[]  UdiffTsProdOutMin=[]  UdiffTsProdOutMax=[]  NTsProdOutMin=[]  NTsProdOutMax=[]  UintegralTsProdOutMin=[]  UintegralTsProdOutMax=[]  UngainTsProdOutMin=[]  UngainTsProdOutMax=[]  ClampingZeroOutDataTypeStr=Inherit: Inherit via back propagation  ClampingZeroOutMin=[]  ClampingZeroOutMax=[]  FilterDenConstantOutDataTypeStr=Inherit: Inherit via back propagation  FilterDenConstantOutMin=[]  FilterDenConstantOutMax=[]  PCopyOutDataTypeStr=Inherit: Inherit via back propagation  PCopyOutMin=[]  PCopyOutMax=[]  NCopyOutDataTypeStr=Inherit: Inherit via back propagation  NCopyOutMin=[]  NCopyOutMax=[]  IntegratorContinuousStateAttributes=''  IntegratorStateMustResolveToSignalObject=off  IntegratorRTWStateStorageClass=Auto  FilterContinuousStateAttributes=''  FilterStateMustResolveToSignalObject=off  FilterRTWStateStorageClass=Auto  ParallelPVariant=InternalParameters  IdealPVariant=Disabled  IVariant=InternalParameters  DVariant=Disabled  IntegratorVariant=Continuous  SatVariant=Enabled  AWVariant=ContClampingParallel  PCopyVariant=Disabled  TRVariant=Disabled  FdbkBlocksVariant=Forward  IdealPFdbkVariant=Disabled  SatFdbkVariant=Disabled  DerivativeFilterVariant=Disabled  NVariant=Disabled  NCopyVariant=Disabled_SignalSpec  FilterICVariant=Disabled  IntegratorICVariant=InternalICs  ExternalResetVariant=ExternalReset  TRSumVariant=Passthrough  SumFdbkVariant=Disabled  SumVariant=Sum_PI  TsampFilterVariant=InternalTs  TsampNgainVariant=Passthrough  TsampIntegralVariant=Disabled_SignalSpec  ExternalSaturationOutDataTypeStr=Inherit: Same as second input
  Radians to Degrees : simulink_extras/Transformations/Radians to Degrees
  Radians to Degrees1 : simulink_extras/Transformations/Radians to Degrees
  Saturation : Saturate  UpperLimit=25/57.3  LowerLimit=-25/57.3
  Scope : Scope
  Scope1 : Scope
  Scope5 : Scope
  Selector1 : Selector  InputPortWidth=3  IndexOptions=Index vector (dialog)  Indices=2  OutputSizes=1
  Selector2 : Selector  InputPortWidth=3  IndexOptions=Index vector (dialog)  Indices=2  OutputSizes=1
  Slon : MultiPortSwitch  Inputs=5  SaturateOnIntegerOverflow=off  InputSameDT=off
  Slon1 : MultiPortSwitch  Inputs=5  SaturateOnIntegerOverflow=off  InputSameDT=off
  "[-15,15]" : Saturate  UpperLimit=15/57.3  LowerLimit=-15/57.3
  "[-15,15]-" : Saturate  UpperLimit=15/57.3  LowerLimit=-15/57.3
  de0 in take-off : Constant  Value=-1.5/57.3
  kq : Gain  Commented=on  Gain=0.5
  kq1 : Gain
  kqi : Gain  Commented=on  Gain=0.02
  kqi2 : Gain  Gain=2
  qc limit : Saturate  UpperLimit=10/57.3  LowerLimit=-10/57.3
  thetac scp : Scope
  de : Outport  VectorParamsAs1DForOutWhenUnconnected=off
  wires:
  Bus Selector1/1 -> [LonMod]  "<LonMod>"
  CMDData/1 -> Bus Selector1/1
  Bus Selector2/2 -> Selector2/1  "<pqr>"
  Selector2/1 -> [q]
  SensorData/1 -> Bus Selector2/1
  thetac/1 -> [thetac]
  Selector1/1 -> [theta]
  Bus Selector2/1 -> Selector1/1  "<Euler>"
  Constant/1 -> Slon1/6
  "[-15,15]-"/1 -> Slon1/5
  [LonMod] -> Slon1/1, Slon/1
  Add2/1 -> OMEGA/1
  [theta] -> Add2/2
  [q] -> Add1/2
  OMEGA/1 -> Scope1/1, qc limit/1
  kq1/1 -> kqi2/1, Slon/4, Slon/3, Slon/2
  de0 in take-off/1 -> Slon/6
  kqi2/1 -> Slon/5
  Memory/1 -> Data Type Conversion/1
  qc limit/1 -> Add1/1  "qc"
  [thetac] -> "[-15,15]-"/1, "[-15,15]"/1
  Radians to Degrees/1 -> thetac scp/1
  "[-15,15]"/1 -> Slon1/4, Slon1/3, Slon1/2
  Integrator/1 -> kqi/1
  Slon1/1 -> Radians to Degrees/1, Memory/1, Add2/1
  Radians to Degrees1/1 -> Scope/1
  Slon/1 -> Saturation/1
  Saturation/1 -> Radians to Degrees1/1, de/1
  kq/1 -> Add4/1
  kqi/1 -> Add4/2
  Add1/1 -> PID Controller/1
  PID Controller/1 -> Scope5/1, kq1/1
  Data Type Conversion/1 -> PID Controller/2

== system eVTOL_PX4_2023b/FCS/FW/trim data ==
  H : Inport
  Gain : Gain  Gain=-0.00000005
  Sum : Sum  Inputs=|+-
  Sum1 : Sum  Inputs=|++
  phic1 : Constant  Value=theta0
  phic2 : Constant  Value=dt0
  phic3 : Constant  Value=h0
  phic9 : Constant  Value=de0
  deTrim : Outport  VectorParamsAs1DForOutWhenUnconnected=off
  dtTrim : Outport  Port=2  VectorParamsAs1DForOutWhenUnconnected=off
  thetaTrim : Outport  Port=3  VectorParamsAs1DForOutWhenUnconnected=off
  wires:
  phic1/1 -> thetaTrim/1
  phic2/1 -> dtTrim/1
  H/1 -> Sum/1
  phic3/1 -> Sum/2
  phic9/1 -> Sum1/2
  Sum1/1 -> deTrim/1
  Sum/1 -> Gain/1
  Gain/1 -> ?

== system eVTOL_PX4_2023b/FCS/MC/ADRC theta ==
  thetac : Inport
  theta : Inport  Port=2
  1/B : Gain  Gain=1/(-125)
  Constant : Constant  Value=[pi/4, 0, 0]
  Demux : Demux  Outputs=3
  ESO : Subsystem
  Gain : Gain  Gain=Kp
  Gain1 : Gain  Gain=Kd
  Mux : Mux  Inputs=2
  Radians to Degrees : simulink_extras/Transformations/Radians to Degrees
  Scope{,1..6} (7 alike) : Scope
  Sum : Sum  Inputs=|+-
  Sum1 : Sum  Inputs=|+-
  Sum2 : Sum  Inputs=|++
  Sum4 : Sum  Inputs=|+-
  TD : Subsystem
  consituous TD : Subsystem
  de : Outport
  wires:
  Demux/2 -> Sum1/2  "theta_dot"
  Sum1/1 -> Gain1/1
  1/B/1 -> Mux/1, de/1, Scope3/1
  theta/1 -> Mux/2
  ESO/1(x) -> ?
  Sum4/1 -> 1/B/1
  Sum2/1 -> Sum4/1  "u0"
  Demux/3 -> Sum4/2  "theta_dotdot"
  ESO/2(y) -> Demux/1
  Gain1/1 -> Scope2/1, Sum2/2
  Demux/1 -> Sum/2  "theta"
  Mux/1 -> ESO/1(u)
  thetac/1 -> consituous TD/1(v), TD/1(v)
  Gain/1 -> Scope1/1, Sum2/1
  Sum/1 -> Gain/1
  Radians to Degrees/1 -> Scope4/1
  Constant/1 -> ESO/2(x0)
  consituous TD/2(v2) -> Sum1/1, Scope/1
  consituous TD/1(v1) -> Sum/1, Radians to Degrees/1
  TD/2(v2) -> Scope5/1
  TD/1(v1) -> Scope6/1

== system eVTOL_PX4_2023b/FCS/MC/Height control ==
  Ve : Inport
  Xe : Inport  Port=2
  h_c : Inport  Port=3
  Demux5 : Demux  Outputs=3
  Demux6 : Demux  Outputs=3
  Gain : Gain  Gain=-1
  Gain4 : Gain  Gain=-1
  Gain5 : Gain  Gain=-1
  PID Controller : slpidlib/PID Controller  Controller=PID  Form=Parallel  TimeDomain=Continuous-time  UseExternalTs=off  SampleTime=-1  IntegratorMethod=Forward Euler  FilterMethod=Forward Euler  ControllerParametersSource=internal  P=0.5  I=0  UseKiTs=off  D=0  N=100  UseFilter=on  TunerSelectOption=Transfer Function Based (PID Tuner App)  InitialConditionSource=internal  InitialConditionForIntegrator=0  InitialConditionForFilter=0  DifferentiatorICPrevScaledInput=0  ExternalReset=none  TrackingMode=off  Kt=1  LimitOutput=off  SatLimitsSource=internal  UpperSaturationLimit=inf  LowerSaturationLimit=-inf  LinearizeAsGain=on  AntiWindupMode=none  Kb=1  LimitIntegrator=off  UpperIntegratorSaturationLimit=inf  LowerIntegratorSaturationLimit=-inf  POutMin=[]  POutMax=[]  IOutMin=[]  IOutMax=[]  DOutMin=[]  DOutMax=[]  NOutMin=[]  NOutMax=[]  SumOutMin=[]  SumOutMax=[]  SaturationOutMin=[]  SaturationOutMax=[]  PParamMin=[]  PParamMax=[]  IParamMin=[]  IParamMax=[]  DParamMin=[]  DParamMax=[]  NParamMin=[]  NParamMax=[]  KbParamMin=[]  KbParamMax=[]  KtParamMin=[]  KtParamMax=[]  KbOutMin=[]  KbOutMax=[]  KtOutMin=[]  KtOutMax=[]  IntegratorOutMin=[]  IntegratorOutMax=[]  FilterOutMin=[]  FilterOutMax=[]  SumI1OutMin=[]  SumI1OutMax=[]  SumI2OutMin=[]  SumI2OutMax=[]  SumI3OutMin=[]  SumI3OutMax=[]  SumI4OutMin=[]  SumI4OutMax=[]  SumDOutMin=[]  SumDOutMax=[]  DifferentiatorOutMin=[]  DifferentiatorOutMax=[]  FilterDiffOutCoefMin=[]  FilterDiffOutCoefMax=[]  ReciprocalOutMin=[]  ReciprocalOutMax=[]  SumDenOutMin=[]  SumDenOutMax=[]  SumNumOutMin=[]  SumNumOutMax=[]  DivideOutMin=[]  DivideOutMax=[]  UdiffTsProdOutMin=[]  UdiffTsProdOutMax=[]  NTsProdOutMin=[]  NTsProdOutMax=[]  UintegralTsProdOutMin=[]  UintegralTsProdOutMax=[]  UngainTsProdOutMin=[]  UngainTsProdOutMax=[]  ClampingZeroOutDataTypeStr=Inherit: Inherit via back propagation  ClampingZeroOutMin=[]  ClampingZeroOutMax=[]  FilterDenConstantOutDataTypeStr=Inherit: Inherit via back propagation  FilterDenConstantOutMin=[]  FilterDenConstantOutMax=[]  PCopyOutDataTypeStr=Inherit: Inherit via back propagation  PCopyOutMin=[]  PCopyOutMax=[]  NCopyOutDataTypeStr=Inherit: Inherit via back propagation  NCopyOutMin=[]  NCopyOutMax=[]  IntegratorContinuousStateAttributes=''  IntegratorStateMustResolveToSignalObject=off  IntegratorRTWStateStorageClass=Auto  FilterContinuousStateAttributes=''  FilterStateMustResolveToSignalObject=off  FilterRTWStateStorageClass=Auto  ParallelPVariant=InternalParameters  IdealPVariant=Disabled  IVariant=InternalParameters  DVariant=InternalParameters  IntegratorVariant=Continuous  SatVariant=Disabled  AWVariant=Passthrough  PCopyVariant=Disabled  TRVariant=Disabled  FdbkBlocksVariant=Forward  IdealPFdbkVariant=Disabled  SatFdbkVariant=Disabled  DerivativeFilterVariant=ContFilter  NVariant=InternalParameters  NCopyVariant=Disabled  FilterICVariant=InternalICsFilter  IntegratorICVariant=InternalICs  ExternalResetVariant=Disabled  TRSumVariant=Passthrough  SumFdbkVariant=Disabled  SumVariant=Sum_PID  TsampFilterVariant=InternalTs  TsampNgainVariant=Passthrough  TsampIntegralVariant=Disabled_SignalSpec  ExternalSaturationOutDataTypeStr=Inherit: Same as second input
  PID Controller2 : slpidlib/PID Controller  Controller=PID  Form=Parallel  TimeDomain=Continuous-time  UseExternalTs=off  SampleTime=-1  IntegratorMethod=Forward Euler  FilterMethod=Forward Euler  ControllerParametersSource=internal  P=1  I=0.3  UseKiTs=off  D=0.1  N=65.6590999771333  UseFilter=on  TunerSelectOption=Transfer Function Based (PID Tuner App)  InitialConditionSource=internal  InitialConditionForIntegrator=0  InitialConditionForFilter=0  DifferentiatorICPrevScaledInput=0  ExternalReset=none  TrackingMode=off  Kt=1  LimitOutput=on  SatLimitsSource=internal  UpperSaturationLimit=1  LowerSaturationLimit=-1  LinearizeAsGain=on  AntiWindupMode=clamping  Kb=1  LimitIntegrator=off  UpperIntegratorSaturationLimit=inf  LowerIntegratorSaturationLimit=-inf  POutMin=[]  POutMax=[]  IOutMin=[]  IOutMax=[]  DOutMin=[]  DOutMax=[]  NOutMin=[]  NOutMax=[]  SumOutMin=[]  SumOutMax=[]  SaturationOutMin=[]  SaturationOutMax=[]  PParamMin=[]  PParamMax=[]  IParamMin=[]  IParamMax=[]  DParamMin=[]  DParamMax=[]  NParamMin=[]  NParamMax=[]  KbParamMin=[]  KbParamMax=[]  KtParamMin=[]  KtParamMax=[]  KbOutMin=[]  KbOutMax=[]  KtOutMin=[]  KtOutMax=[]  IntegratorOutMin=[]  IntegratorOutMax=[]  FilterOutMin=[]  FilterOutMax=[]  SumI1OutMin=[]  SumI1OutMax=[]  SumI2OutMin=[]  SumI2OutMax=[]  SumI3OutMin=[]  SumI3OutMax=[]  SumI4OutMin=[]  SumI4OutMax=[]  SumDOutMin=[]  SumDOutMax=[]  DifferentiatorOutMin=[]  DifferentiatorOutMax=[]  FilterDiffOutCoefMin=[]  FilterDiffOutCoefMax=[]  ReciprocalOutMin=[]  ReciprocalOutMax=[]  SumDenOutMin=[]  SumDenOutMax=[]  SumNumOutMin=[]  SumNumOutMax=[]  DivideOutMin=[]  DivideOutMax=[]  UdiffTsProdOutMin=[]  UdiffTsProdOutMax=[]  NTsProdOutMin=[]  NTsProdOutMax=[]  UintegralTsProdOutMin=[]  UintegralTsProdOutMax=[]  UngainTsProdOutMin=[]  UngainTsProdOutMax=[]  ClampingZeroOutDataTypeStr=Inherit: Inherit via back propagation  ClampingZeroOutMin=[]  ClampingZeroOutMax=[]  FilterDenConstantOutDataTypeStr=Inherit: Inherit via back propagation  FilterDenConstantOutMin=[]  FilterDenConstantOutMax=[]  PCopyOutDataTypeStr=Inherit: Inherit via back propagation  PCopyOutMin=[]  PCopyOutMax=[]  NCopyOutDataTypeStr=Inherit: Inherit via back propagation  NCopyOutMin=[]  NCopyOutMax=[]  IntegratorContinuousStateAttributes=''  IntegratorStateMustResolveToSignalObject=off  IntegratorRTWStateStorageClass=Auto  FilterContinuousStateAttributes=''  FilterStateMustResolveToSignalObject=off  FilterRTWStateStorageClass=Auto  ParallelPVariant=InternalParameters  IdealPVariant=Disabled  IVariant=InternalParameters  DVariant=InternalParameters  IntegratorVariant=Continuous  SatVariant=Enabled  AWVariant=ContClampingParallel  PCopyVariant=Disabled  TRVariant=Disabled  FdbkBlocksVariant=Forward  IdealPFdbkVariant=Disabled  SatFdbkVariant=Disabled  DerivativeFilterVariant=ContFilter  NVariant=InternalParameters  NCopyVariant=Disabled  FilterICVariant=InternalICsFilter  IntegratorICVariant=InternalICs  ExternalResetVariant=Disabled  TRSumVariant=Passthrough  SumFdbkVariant=Disabled  SumVariant=Sum_PID  TsampFilterVariant=InternalTs  TsampNgainVariant=Passthrough  TsampIntegralVariant=Disabled_SignalSpec  ExternalSaturationOutDataTypeStr=Inherit: Same as second input
  Saturation1 : Saturate  UpperLimit=2.5  LowerLimit=-2.5
  Scope : Scope  NumInputPorts=2
  Scope1 : Scope  NumInputPorts=2
  Scope2 : Scope
  Sum1 : Sum  Inputs=|-+
  Sum4 : Sum  Inputs=|-+
  Terminator{,1..3} (4 alike) : Terminator
  dt : Outport
  wires:
  Demux6/3 -> Sum1/1, Gain5/1
  h_c/1 -> Scope1/2, Gain/1
  Ve/1 -> Demux5/1
  Demux5/2 -> Terminator1/1
  Demux6/1 -> Terminator2/1
  Demux5/1 -> Terminator/1
  Xe/1 -> Demux6/1
  Demux5/3 -> Sum4/1, Scope/1  "Vz"
  Sum1/1 -> PID Controller/1
  Demux6/2 -> Terminator3/1
  Gain/1 -> Sum1/2
  PID Controller/1 -> Saturation1/1  "Vzc"
  Gain5/1 -> Scope1/1  "h"
  PID Controller2/1 -> Gain4/1, Scope2/1
  Sum4/1 -> PID Controller2/1
  Gain4/1 -> dt/1
  Saturation1/1 -> Sum4/2, Scope/2  "Vz_c"
